simulink library "LopesDevelopmentLibrary"  (R2015b)
settings: Solver=ode45  StartTime=0.0  StopTime=10.0  RelTol=1e-3
values from neighbouring files (symbols this model uses):
  d2r = @(d) d*(pi/180)    [LopesDevelopmentLibrary_LoadParameters.m]
  ts = LopesParams.ts    [LopesDevelopmentLibrary_LoadParameters.m]
undefined symbols (not defined in the file or in its folder): anyParameterChanged, DiscIntNeverNeededParam, gcbh, LHF, LKF, LopesParams, macaddr, mxpcnetworkconfig, mxpcrtudprx, mxpcrtudptx, patientParametersChanged, port, PX, PZ, RHF, RKF, SelectorLOPESInSize, StrideTime_s, Time
undefined symbols (not defined in the file): LopesParamsSendDataArrayLen
libraries: LopesDevelopmentLibrary x288, simulink x98, dspmtrx3 x47, xpciplib x6, xpcnetworkbufferlib x5, dspsigops x4, dspstat3 x3, xpcethernetlib x2, visionstatistics x2, xpcseriallib x2, nmc x1, simulink_extras x1
(part 9 of 12)

== system LopesDevelopmentLibrary/GaitGenerationExtra/CalculateBreaksCoefs/Calculate/RightHipFlexion1 ==
  parameters : Inport
  HipExtensionOffset_pct : Inport  Port=2
  Steplength_Length_pct : Inport  Port=3
  SteplengthOtherLeg_Length_pct : Inport  Port=4
  StepHeight_KneeFlexion_pct : Inport  Port=5
  AddToMatrixColumn : LopesDevelopmentLibrary/Various/AddToMatrixColumn  col=2  minimum=-inf  maximum=inf
  Bias : Bias  Bias=100
  Bias1 : Bias  Bias=100
  Gain1 : Gain  Gain=1/100
  Gain2 : Gain  Gain=1/100
  Gain3 : Gain  Gain=0.01* d2r(2.5)
  Gain4 : Gain  Gain=0.01* d2r(5)
  GainHipExtensionOffset : Gain  Gain=-0.01* d2r(10)
  KneeFlexionStepheight : LopesDevelopmentLibrary/Various/AddToMatrixElement  row=5  col=2  minimum=0  maximum=d2r(90)
  KneeFlexionStepheight1 : LopesDevelopmentLibrary/Various/AddToMatrixElement  row=6  col=2  minimum=0  maximum=d2r(90)
  MultiplyMatrixElement : LopesDevelopmentLibrary/Various/MultiplyMatrixElement  row=6  col=2  minimum=-inf  maximum=inf
  MultiplyMatrixElement1 : LopesDevelopmentLibrary/Various/MultiplyMatrixElement  row=4  col=2  minimum=-inf  maximum=inf
  MultiplyMatrixElement2 : LopesDevelopmentLibrary/Various/MultiplyMatrixElement  row=1  col=2  minimum=-inf  maximum=inf
  MultiplyMatrixElement3 : LopesDevelopmentLibrary/Various/MultiplyMatrixElement  row=2  col=2  minimum=-inf  maximum=inf
  RatioFlexionExtension : Gain
  RegressionData : Constant  Value=LopesParams.GaitData.RHF
  RegressionData2KeyEvents : LopesDevelopmentLibrary/BlocksForInternalUse/GaitGeneration/RegressionData2KeyEvents
  KeyEvents : Outport
  wires:
  MultiplyMatrixElement1/1 -> KeyEvents/1
  AddToMatrixColumn/1 -> MultiplyMatrixElement/1
  Gain2/1 -> MultiplyMatrixElement1/2
  Steplength_Length_pct/1 -> Bias/1
  Bias/1 -> Gain1/1
  Gain1/1 -> MultiplyMatrixElement3/2, MultiplyMatrixElement2/2, MultiplyMatrixElement/2
  Bias1/1 -> Gain2/1
  SteplengthOtherLeg_Length_pct/1 -> RatioFlexionExtension/1
  RegressionData/1 -> RegressionData2KeyEvents/1
  parameters/1 -> RegressionData2KeyEvents/2
  KneeFlexionStepheight/1 -> KneeFlexionStepheight1/1
  RegressionData2KeyEvents/1 -> KneeFlexionStepheight/1
  Gain3/1 -> KneeFlexionStepheight/2
  Gain4/1 -> KneeFlexionStepheight1/2
  StepHeight_KneeFlexion_pct/1 -> Gain4/1, Gain3/1
  HipExtensionOffset_pct/1 -> GainHipExtensionOffset/1
  KneeFlexionStepheight1/1 -> AddToMatrixColumn/1
  GainHipExtensionOffset/1 -> AddToMatrixColumn/2
  RatioFlexionExtension/1 -> Bias1/1
  MultiplyMatrixElement/1 -> MultiplyMatrixElement2/1
  MultiplyMatrixElement2/1 -> MultiplyMatrixElement3/1
  MultiplyMatrixElement3/1 -> MultiplyMatrixElement1/1

== system LopesDevelopmentLibrary/GaitGenerationExtra/CalculateBreaksCoefs/Calculate/RightKneeFlexion1 ==
  parameters : Inport
  StepHeight_KneeFlexion_pct : Inport  Port=2
  Prepositioning_KneeFlexion_pct : Inport  Port=3
  StabilityStance_Kneeflexion_pct : Inport  Port=4
  StepLength_pct : Inport  Port=5
  Constant : Constant  Value=-inf
  Gain1 : Gain  Gain=0.01* d2r(5)
  Gain2 : Gain  Gain=0.01* d2r(10)
  Gain3 : Gain  Gain=0.01* d2r(5)
  Gain4 : Gain  Gain=0.01* d2r(20)
  Gain5 : Gain  Gain=-0.01/3
  KneeFlexionPrepositioning : LopesDevelopmentLibrary/Various/AddToMatrixElement  row=1  col=2  minimum=0  maximum=d2r(90)
  KneefFlexionStepheigh : LopesDevelopmentLibrary/Various/AddToMatrixElement  row=5  col=2  minimum=0  maximum=d2r(90)
  KneefFlexionStepheigh1 : LopesDevelopmentLibrary/Various/AddToMatrixElement  row=6  col=2  minimum=0  maximum=d2r(90)
  KneeflexionStance : LopesDevelopmentLibrary/Various/AddToMatrixElement  row=2  col=2  minimum=0  maximum=d2r(90)
  RatioKey6toKey1 : Gain  Gain=1/2
  RegressionData : Constant  Value=LopesParams.GaitData.RKF
  RegressionData2KeyEvents : LopesDevelopmentLibrary/BlocksForInternalUse/GaitGeneration/RegressionData2KeyEvents
  Saturation : Saturate  UpperLimit=0  LowerLimit=-inf
  Saturation Dynamic : simulink/Discontinuities/Saturation Dynamic  OutMin=[]  OutMax=[]  OutDataTypeStr=Inherit: Same as second input  OutDataType=fixdt(1, 16)  OutScaling=2^-10  DoSatur=off
  SelectorK1 : Selector  NumberOfDimensions=2  InputPortWidth=3  IndexOptions=Index vector (dialog),Index vector (dialog)  Indices=1,2  OutputSizes=1,1
  SelectorK2 : Selector  NumberOfDimensions=2  InputPortWidth=3  IndexOptions=Index vector (dialog),Index vector (dialog)  Indices=2,2  OutputSizes=1,1
  Steplength1 : LopesDevelopmentLibrary/Various/AddToMatrixElement  row=1  col=2  minimum=0  maximum=d2r(90)
  Steplength2 : LopesDevelopmentLibrary/Various/AddToMatrixElement  row=6  col=2  minimum=0  maximum=d2r(90)
  Sum : Sum  Inputs=++|
  Sum1 : Sum  Inputs=-+|
  KeyEvents : Outport
  wires:
  Gain4/1 -> KneefFlexionStepheigh1/2
  KneefFlexionStepheigh1/1 -> KneeFlexionPrepositioning/1
  Gain3/1 -> KneeflexionStance/2
  Gain2/1 -> KneefFlexionStepheigh/2
  StepHeight_KneeFlexion_pct/1 -> Gain2/1, Gain4/1
  KneefFlexionStepheigh/1 -> KneefFlexionStepheigh1/1
  RegressionData2KeyEvents/1 -> KneefFlexionStepheigh/1
  KneeFlexionPrepositioning/1 -> KneeflexionStance/1
  parameters/1 -> RegressionData2KeyEvents/2
  RegressionData/1 -> RegressionData2KeyEvents/1
  Prepositioning_KneeFlexion_pct/1 -> Gain1/1
  StabilityStance_Kneeflexion_pct/1 -> Gain3/1
  Gain1/1 -> KneeFlexionPrepositioning/2
  StepLength_pct/1 -> Saturation/1
  Steplength1/1 -> Steplength2/1
  RatioKey6toKey1/1 -> Steplength2/2
  SelectorK2/1 -> Saturation Dynamic/1
  Constant/1 -> Saturation Dynamic/3
  SelectorK1/1 -> Sum1/1, Sum/1
  Gain5/1 -> Sum/2
  Sum/1 -> Saturation Dynamic/2
  Sum1/1 -> RatioKey6toKey1/1, Steplength1/2
  Saturation Dynamic/1 -> Sum1/2
  Saturation/1 -> Gain5/1
  Steplength2/1 -> KeyEvents/1
  KneeflexionStance/1 -> SelectorK1/1, SelectorK2/1, Steplength1/1

== system LopesDevelopmentLibrary/GaitGenerationExtra/CalculateBreaksCoefs/Calculate/Time1 ==
  note: v = strideLengh * nStridesPerSecond
      |                   = strideLength / nSecondsPerStride
      | strideTime = nSecondsPerStride = strideLength / v
  note: The key event matrix is generated here; it consists
      | of two rows (ie, a key event at 0% and one at 100%),
      | and the start time (=0) and end time. We need to
      | calculate the slope (in s/%) as well to get a straight line.
  WalkingVelocity_m_s : Inport
  BreaksCoefsBus : Inport  Port=2
  Parameters : Inport  Port=3
  CalculateStrideLength : Subsystem
  Constant : Constant  Value=[0,0,nan; 100,nan,nan]
  Gain : Gain  Gain=0.01
  Mux : Mux  Inputs=2
  Overwrite Values : dspmtrx3/Overwrite Values  OverWriteDiag=Submatrix  valFrom2ndIP=Second input port  ConstValue=0  RowSpan=One row  RowStartMode=Index  RowStartIndex=2  RowEndMode=Last  RowEndIndex=1  ColSpan=One column  ColStartMode=Index  ColStartIndex=2  ColEndMode=Last  ColEndIndex=1  DiagSpan=Range of elements  DiagStartMode=Index  DiagStartIndex=2  DiagEndMode=Index  DiagEndIndex=4
  Overwrite Values1 : dspmtrx3/Overwrite Values  OverWriteDiag=Submatrix  valFrom2ndIP=Second input port  ConstValue=0  RowSpan=All rows  RowStartMode=Index  RowStartIndex=2  RowEndMode=Last  RowEndIndex=1  ColSpan=One column  ColStartMode=Last  ColStartIndex=2  ColEndMode=Last  ColEndIndex=1  DiagSpan=Range of elements  DiagStartMode=Index  DiagStartIndex=2  DiagEndMode=Index  DiagEndIndex=4
  SafeDivide : LopesDevelopmentLibrary/Various/SafeDivide  SystemSampleTime=-1
  KeyEvents : Outport
  StrideTime_s : Outport  Port=2
  wires:
  Mux/1 -> Overwrite Values1/2
  Overwrite Values/1 -> Overwrite Values1/1
  Gain/1 -> Mux/2, Mux/1  "slope"
  Constant/1 -> Overwrite Values/1
  SafeDivide/1 -> StrideTime_s/1, Gain/1, Overwrite Values/2  "StrideTime"
  Overwrite Values1/1 -> KeyEvents/1
  BreaksCoefsBus/1 -> CalculateStrideLength/1(BreaksCoefsBus)
  Parameters/1 -> CalculateStrideLength/2(Parameters)
  WalkingVelocity_m_s/1 -> SafeDivide/2
  CalculateStrideLength/1(StrideLength) -> SafeDivide/1

== system LopesDevelopmentLibrary/GaitGenerationExtra/CalculateBreaksCoefs/Calculate/Unactuated DOFS ==

== system LopesDevelopmentLibrary/GaitGenerationExtra/PhaseEstimatorAoyagi_wPI_Extra/EstimatePhaseDirectlyAoyagi/CalculateFullReferenceTrajectory ==
  BreaksCoefs : Inport
  xx : Inport  Port=2
  Enable : EnablePort
  Bus Selector2 : BusSelector  OutputSignals=LHF,LKF,RHF,RKF,StrideTime_s
  Divide{,1,3..4} (4 alike) : Product  Inputs=*/
  Gain : Gain  Gain=0.01
  Terminator{,1,3..4} (4 alike) : Terminator
  ppval_bus_LHF : LopesDevelopmentLibrary/BlocksForInternalUse/GaitGeneration/ppval_bus
  ppval_bus_LKF : LopesDevelopmentLibrary/BlocksForInternalUse/GaitGeneration/ppval_bus
  ppval_bus_RHF : LopesDevelopmentLibrary/BlocksForInternalUse/GaitGeneration/ppval_bus
  ppval_bus_RKF : LopesDevelopmentLibrary/BlocksForInternalUse/GaitGeneration/ppval_bus
  LHF_yy : Outport
  LKF_yy : Outport  Port=2
  RHF_yy : Outport  Port=3
  RKF_yy : Outport  Port=4
  LHF_dydt : Outport  Port=5
  LKF_dydt : Outport  Port=6
  RHF_dydt : Outport  Port=7
  RKF_dydt : Outport  Port=8
  wires:
  xx/1 -> ppval_bus_RHF/1, ppval_bus_RKF/1, ppval_bus_LKF/1, ppval_bus_LHF/1
  BreaksCoefs/1 -> Bus Selector2/1
  ppval_bus_RHF/3 -> Terminator3/1
  ppval_bus_LKF/3 -> Terminator1/1
  ppval_bus_RKF/3 -> Terminator4/1
  ppval_bus_LHF/3 -> Terminator/1
  Divide4/1 -> RKF_dydt/1
  Divide3/1 -> RHF_dydt/1
  Divide1/1 -> LKF_dydt/1
  Divide/1 -> LHF_dydt/1
  Gain/1 -> Divide/2, Divide1/2, Divide3/2, Divide4/2  "dtdx"
  ppval_bus_RKF/2 -> Divide4/1
  ppval_bus_RHF/2 -> Divide3/1
  ppval_bus_LKF/2 -> Divide1/1
  ppval_bus_LHF/2 -> Divide/1
  ppval_bus_RKF/1 -> RKF_yy/1
  ppval_bus_RHF/1 -> RHF_yy/1
  Bus Selector2/1 -> ppval_bus_LHF/2  "<LHF>"
  Bus Selector2/2 -> ppval_bus_LKF/2  "<LKF>"
  Bus Selector2/3 -> ppval_bus_RHF/2  "<RHF>"
  Bus Selector2/4 -> ppval_bus_RKF/2  "<RKF>"
  Bus Selector2/5 -> Gain/1  "<StrideTime_s>"
  ppval_bus_LHF/1 -> LHF_yy/1
  ppval_bus_LKF/1 -> LKF_yy/1

== system LopesDevelopmentLibrary/GaitGenerationExtra/PhaseEstimatorAoyagi_wPI_Extra/PhaseFilterAoyagi/FinalStateFinisher ==
  note: This block is implemented to have a minimum PhasePercRate during the last step
      | In this way, the last step is always finalized
  PhasePercRate : Inport
  FinalState : Inport  Port=2
  Constant : Constant  Value=inf
  Constant1 : Constant  Value=20
  Product : Product  OutDataTypeStr=double
  Saturation : simulink/Discontinuities/Saturation Dynamic  OutMin=[]  OutMax=[]  OutDataTypeStr=Inherit: Same as second input  OutDataType=fixdt(1, 16)  OutScaling=2^-10  DoSatur=off
  PhasePercRateOut : Outport
  wires:
  PhasePercRate/1 -> Saturation/2
  Constant/1 -> Saturation/1
  Constant1/1 -> Product/1
  FinalState/1 -> Product/2
  Saturation/1 -> PhasePercRateOut/1
  Product/1 -> Saturation/3

== system LopesDevelopmentLibrary/GaitGenerationExtra/PhaseEstimatorAoyagi_wPI_Extra/PhaseFilterAoyagi/Wrap_Min50_Plus50 ==
  note: Wraps the input phase such
      | that the output is always
      | in the range -50<=out<50
      | (even if input is negative).
  In : Inport
  Bias : Bias  Bias=50
  Bias1 : Bias  Bias=-50
  Constant1 : Constant  Value=100
  ShiftedPhase1 : Math  Operator=mod  SaturateOnIntegerOverflow=on
  Out : Outport
  wires:
  Bias1/1 -> Out/1
  Bias/1 -> ShiftedPhase1/1
  Constant1/1 -> ShiftedPhase1/2
  In/1 -> Bias/1
  ShiftedPhase1/1 -> Bias1/1

== system LopesDevelopmentLibrary/GaitPhaseDetection/Gait Phase Detection with Wrapper/Data selection/Angle_l ==
  ankle : Inport
  knee : Inport  Port=2
  hip : Inport  Port=3
  Dot Product : DotProduct  InputSameDT=on  OutDataTypeStr=Inherit: Inherit via internal rule
  Sum1 : Sum  Inputs=-+
  Sum2 : Sum  Inputs=+-
  Trigonometric Function : Trigonometry  Operator=acos
  angle_l : Outport
  wires:
  Sum2/1 -> Dot Product/1
  ankle/1 -> Sum2/1
  Sum1/1 -> Dot Product/2
  hip/1 -> Sum1/2
  knee/1 -> Sum2/2, Sum1/1
  Dot Product/1 -> Trigonometric Function/1
  Trigonometric Function/1 -> angle_l/1

== system LopesDevelopmentLibrary/GaitPhaseDetection/Gait Phase Detection with Wrapper/Data selection/Angle_r ==
  ankle : Inport
  knee : Inport  Port=2
  hip : Inport  Port=3
  Dot Product : DotProduct  InputSameDT=on  OutDataTypeStr=Inherit: Inherit via internal rule
  Sum1 : Sum  Inputs=-+
  Sum2 : Sum  Inputs=+-
  Trigonometric Function : Trigonometry  Operator=acos
  angle_r : Outport
  wires:
  Trigonometric Function/1 -> angle_r/1
  Dot Product/1 -> Trigonometric Function/1
  knee/1 -> Sum1/1, Sum2/2
  hip/1 -> Sum1/2
  Sum1/1 -> Dot Product/2
  ankle/1 -> Sum2/1
  Sum2/1 -> Dot Product/1

== system LopesDevelopmentLibrary/GaitPhaseDetection/Gait Phase Detection with Wrapper/LeftLegWalking/Heel strike detection ==
  note: DAL (daling voor stijging)
  ankle_y_dot : Inport
  ankle_x_dot : Inport  Port=2
  " " : simulink/Logic and Bit Operations/Compare To Constant  relop===  const=0  OutDataTypeStr=uint8  ZeroCross=off
  "   " : MinMax
  "        " : simulink/Discrete/Tapped Delay  vinit=0.0  samptime=-1  NumDelays=5  DelayOrder=Oldest  includeCurrent=off
  "               " : DataTypeConversion
  Daldetectie_stijging : simulink/Logic and Bit Operations/Detect Increase  vinit=0.0  InputProcessing=Inherited  OutDataTypeStr=uint8
  Logical Operator : Logic  Inputs=3  AllPortsSameDT=off  OutDataTypeStr=boolean
  Voorwaarde voor stap_3 : simulink/Logic and Bit Operations/Compare To Constant  relop=<  const=0  OutDataTypeStr=uint8  ZeroCross=off
  Heel_strike : Outport
  wires:
  "   "/1 -> " "/1
  "        "/1 -> "   "/1
  Voorwaarde voor stap_3/1 -> Logical Operator/3
  "               "/1 -> "        "/1
  Daldetectie_stijging/1 -> "               "/1, Logical Operator/1
  Logical Operator/1 -> Heel_strike/1
  ankle_y_dot/1 -> Daldetectie_stijging/1
  ankle_x_dot/1 -> Voorwaarde voor stap_3/1
  " "/1 -> Logical Operator/2

== system LopesDevelopmentLibrary/GaitPhaseDetection/Gait Phase Detection with Wrapper/LeftLegWalking/Heel strike_safety ==
  ankle_x_dot : Inport
  belt_speed : Inport  Port=2
  "        " : simulink/Discrete/Tapped Delay  vinit=0  samptime=-1  NumDelays=20  DelayOrder=Oldest  includeCurrent=off
  2-D Mean : visionstatistics/2-D Mean  run=off  reset_popup=None  directionMode=Entire input  dimension=1  treatSBRowAsCol=on  roiEnable=off  roiType=Rectangles  roiPortion=Entire ROI  roiOutput=Individual statistics for each ROI  roiFlag=off  outputDataTypeStr=Inherit: Same as accumulator  outputLastDataTypeStr=Inherit: Same as accumulator  outputMin=[]  outputMax=[]  accumMode=Binary point scaling  accumWordLength=32  accumFracLength=0  accumDataTypeStr=fixdt([],32,0)  accumLastDataTypeStr=fixdt([],32,0)  roundingMode=Floor  overflowMode=off
  Daldetectie_stijging2 : simulink/Logic and Bit Operations/Detect Increase  vinit=0.0  InputProcessing=Inherited  OutDataTypeStr=uint8
  Data Type Conversion2 : DataTypeConversion
  Gain2 : Gain  Gain=-0.95
  Relational Operator : RelationalOperator  Operator=<  OutDataTypeStr=boolean
  Heel_strike_safety : Outport
  wires:
  belt_speed/1 -> Gain2/1
  ankle_x_dot/1 -> "        "/1
  "        "/1 -> 2-D Mean/1
  Relational Operator/1 -> Data Type Conversion2/1
  Data Type Conversion2/1 -> Daldetectie_stijging2/1
  Daldetectie_stijging2/1 -> Heel_strike_safety/1
  2-D Mean/1 -> Relational Operator/1
  Gain2/1 -> Relational Operator/2

== system LopesDevelopmentLibrary/GaitPhaseDetection/Gait Phase Detection with Wrapper/LeftLegWalking/Toe-off detection ==
  ankle_x_dot : Inport
  knee_angle_dot : Inport  Port=2
  Daldetectie_stijging1 : simulink/Logic and Bit Operations/Detect Increase  vinit=0.0  InputProcessing=Inherited  OutDataTypeStr=uint8
  Daldetectie_stijging2 : simulink/Logic and Bit Operations/Detect Increase  vinit=0.0  InputProcessing=Inherited  OutDataTypeStr=uint8
  Data Type Conversion1 : DataTypeConversion
  Gain : Gain  Gain=2
  Logical Operator : Logic  AllPortsSameDT=off  OutDataTypeStr=boolean
  Voorwaarde voor stap_4 : simulink/Logic and Bit Operations/Compare To Constant  relop=>  const=0  OutDataTypeStr=uint8  ZeroCross=off
  Toe_off : Outport
  wires:
  Daldetectie_stijging1/1 -> Gain/1
  Logical Operator/1 -> Data Type Conversion1/1
  Data Type Conversion1/1 -> Daldetectie_stijging1/1
  Voorwaarde voor stap_4/1 -> Logical Operator/1
  Gain/1 -> Toe_off/1
  knee_angle_dot/1 -> Daldetectie_stijging2/1
  Daldetectie_stijging2/1 -> Logical Operator/2
  ankle_x_dot/1 -> Voorwaarde voor stap_4/1

== system LopesDevelopmentLibrary/GaitPhaseDetection/Gait Phase Detection with Wrapper/RightLegWalking/Heel strike detection ==
  note: DAL (daling voor stijging)
  ankle_y_dot : Inport
  ankle_x_dot : Inport  Port=2
  " " : simulink/Logic and Bit Operations/Compare To Constant  relop===  const=0  OutDataTypeStr=uint8  ZeroCross=off
  "   " : MinMax
  "        " : simulink/Discrete/Tapped Delay  vinit=0.0  samptime=-1  NumDelays=5  DelayOrder=Oldest  includeCurrent=off
  "               " : DataTypeConversion
  Daldetectie_stijging : simulink/Logic and Bit Operations/Detect Increase  vinit=0.0  InputProcessing=Inherited  OutDataTypeStr=uint8
  Logical Operator : Logic  Inputs=3  AllPortsSameDT=off  OutDataTypeStr=boolean
  Voorwaarde voor stap_3 : simulink/Logic and Bit Operations/Compare To Constant  relop=<  const=0  OutDataTypeStr=uint8  ZeroCross=off
  Heel_strike : Outport
  wires:
  Daldetectie_stijging/1 -> Logical Operator/1, "               "/1
  "               "/1 -> "        "/1
  Voorwaarde voor stap_3/1 -> Logical Operator/3
  "        "/1 -> "   "/1
  "   "/1 -> " "/1
  Logical Operator/1 -> Heel_strike/1
  ankle_y_dot/1 -> Daldetectie_stijging/1
  ankle_x_dot/1 -> Voorwaarde voor stap_3/1
  " "/1 -> Logical Operator/2

== system LopesDevelopmentLibrary/GaitPhaseDetection/Gait Phase Detection with Wrapper/RightLegWalking/Heel strike_safety ==
  ankle_x_dot : Inport
  belt_speed : Inport  Port=2
  "        " : simulink/Discrete/Tapped Delay  vinit=0  samptime=-1  NumDelays=20  DelayOrder=Oldest  includeCurrent=off
  2-D Mean : visionstatistics/2-D Mean  run=off  reset_popup=None  directionMode=Entire input  dimension=1  treatSBRowAsCol=on  roiEnable=off  roiType=Rectangles  roiPortion=Entire ROI  roiOutput=Individual statistics for each ROI  roiFlag=off  outputDataTypeStr=Inherit: Same as accumulator  outputLastDataTypeStr=Inherit: Same as accumulator  outputMin=[]  outputMax=[]  accumMode=Binary point scaling  accumWordLength=32  accumFracLength=0  accumDataTypeStr=fixdt([],32,0)  accumLastDataTypeStr=fixdt([],32,0)  roundingMode=Floor  overflowMode=off
  Daldetectie_stijging2 : simulink/Logic and Bit Operations/Detect Increase  vinit=0.0  InputProcessing=Inherited  OutDataTypeStr=uint8
  Data Type Conversion2 : DataTypeConversion
  Gain2 : Gain  Gain=-0.95
  Relational Operator : RelationalOperator  Operator=<  OutDataTypeStr=boolean
  Heel_strike_safety : Outport
  wires:
  Daldetectie_stijging2/1 -> Heel_strike_safety/1
  Data Type Conversion2/1 -> Daldetectie_stijging2/1
  Relational Operator/1 -> Data Type Conversion2/1
  "        "/1 -> 2-D Mean/1
  ankle_x_dot/1 -> "        "/1
  2-D Mean/1 -> Relational Operator/1
  belt_speed/1 -> Gain2/1
  Gain2/1 -> Relational Operator/2

== system LopesDevelopmentLibrary/GaitPhaseDetection/Gait Phase Detection with Wrapper/RightLegWalking/Toe-off detection ==
  ankle_x_dot : Inport
  knee_angle_dot : Inport  Port=2
  Daldetectie_stijging1 : simulink/Logic and Bit Operations/Detect Increase  vinit=0.0  InputProcessing=Inherited  OutDataTypeStr=uint8
  Daldetectie_stijging2 : simulink/Logic and Bit Operations/Detect Increase  vinit=0.0  InputProcessing=Inherited  OutDataTypeStr=uint8
  Data Type Conversion1 : DataTypeConversion
  Gain : Gain  Gain=2
  Logical Operator : Logic  AllPortsSameDT=off  OutDataTypeStr=boolean
  Voorwaarde voor stap_4 : simulink/Logic and Bit Operations/Compare To Constant  relop=>  const=0  OutDataTypeStr=uint8  ZeroCross=off
  Toe_off : Outport
  wires:
  Voorwaarde voor stap_4/1 -> Logical Operator/1
  Data Type Conversion1/1 -> Daldetectie_stijging1/1
  Gain/1 -> Toe_off/1
  knee_angle_dot/1 -> Daldetectie_stijging2/1
  Logical Operator/1 -> Data Type Conversion1/1
  Daldetectie_stijging1/1 -> Gain/1
  Daldetectie_stijging2/1 -> Logical Operator/2
  ankle_x_dot/1 -> Voorwaarde voor stap_4/1

== system LopesDevelopmentLibrary/GaitPhaseDetection/Gait Phase Detection with Wrapper/Smart derivative/Filtered derivative ==
  note: This block is a derivative function
      | second order low pass filter with
      | settable zeta and omega.
      | It works for scalars as well as vectors.
      |
      | You can monitor the output from Python
      | by monitoring OutputValue.s[0,:]
  x : Inport
  cut-off (hz) : Inport  Port=2
  Discrete-Time Integrator : DiscreteIntegrator  InitialConditionSetting=State (most efficient)  SampleTime=-1  ICPrevOutput=DiscIntNeverNeededParam  ICPrevScaledInput=DiscIntNeverNeededParam
  Discrete-Time Integrator1 : DiscreteIntegrator  InitialConditionSetting=State (most efficient)  SampleTime=-1  ICPrevOutput=DiscIntNeverNeededParam  ICPrevScaledInput=DiscIntNeverNeededParam
  Gain : Gain  Gain=2*pi
  Product1 : Product  RndMeth=Zero
  Product2 : Product  RndMeth=Zero
  Sum : Sum  Inputs=|+-
  Sum1 : Sum  Inputs=|+-
  omega_sq : Math  Operator=square  SaturateOnIntegerOverflow=on
  two : Constant  Value=2
  zeta : Constant  Value=0.7
  zeta_omega_2 : Product  Inputs=3  RndMeth=Zero
  x_dot : Outport
  wires:
  Discrete-Time Integrator1/1 -> Sum/2
  Product2/1 -> Sum1/2
  zeta_omega_2/1 -> Product2/2
  Product1/1 -> Sum1/1
  Discrete-Time Integrator/1 -> Discrete-Time Integrator1/1, x_dot/1, Product2/1
  two/1 -> zeta_omega_2/1
  Sum/1 -> Product1/1
  cut-off (hz)/1 -> Gain/1
  zeta/1 -> zeta_omega_2/2
  omega_sq/1 -> Product1/2
  x/1 -> Sum/1
  Sum1/1 -> Discrete-Time Integrator/1
  Gain/1 -> omega_sq/1, zeta_omega_2/3

== system LopesDevelopmentLibrary/GaitPhaseDetection/Gait Phase Detection with Wrapper/Smart derivative/Filtered derivative1 ==
  note: This block is a derivative function
      | second order low pass filter with
      | settable zeta and omega.
      | It works for scalars as well as vectors.
      |
      | You can monitor the output from Python
      | by monitoring OutputValue.s[0,:]
  x : Inport
  cut-off (hz) : Inport  Port=2
  Discrete-Time Integrator : DiscreteIntegrator  InitialConditionSetting=State (most efficient)  SampleTime=-1  ICPrevOutput=DiscIntNeverNeededParam  ICPrevScaledInput=DiscIntNeverNeededParam
  Discrete-Time Integrator1 : DiscreteIntegrator  InitialConditionSetting=State (most efficient)  SampleTime=-1  ICPrevOutput=DiscIntNeverNeededParam  ICPrevScaledInput=DiscIntNeverNeededParam
  Gain : Gain  Gain=2*pi
  Product1 : Product  RndMeth=Zero
  Product2 : Product  RndMeth=Zero
  Sum : Sum  Inputs=|+-
  Sum1 : Sum  Inputs=|+-
  omega_sq : Math  Operator=square  SaturateOnIntegerOverflow=on
  two : Constant  Value=2
  zeta : Constant  Value=0.7
  zeta_omega_2 : Product  Inputs=3  RndMeth=Zero
  x_dot : Outport
  wires:
  Gain/1 -> zeta_omega_2/3, omega_sq/1
  Sum1/1 -> Discrete-Time Integrator/1
  x/1 -> Sum/1
  omega_sq/1 -> Product1/2
  zeta/1 -> zeta_omega_2/2
  cut-off (hz)/1 -> Gain/1
  Sum/1 -> Product1/1
  two/1 -> zeta_omega_2/1
  Discrete-Time Integrator/1 -> Product2/1, x_dot/1, Discrete-Time Integrator1/1
  Product1/1 -> Sum1/1
  zeta_omega_2/1 -> Product2/2
  Product2/1 -> Sum1/2
  Discrete-Time Integrator1/1 -> Sum/2

== system LopesDevelopmentLibrary/GaitPhaseDetection/Gait Phase Detection with Wrapper/Smart derivative/Filtered derivative2 ==
  note: This block is a derivative function
      | second order low pass filter with
      | settable zeta and omega.
      | It works for scalars as well as vectors.
      |
      | You can monitor the output from Python
      | by monitoring OutputValue.s[0,:]
  x : Inport
  cut-off (hz) : Inport  Port=2
  Discrete-Time Integrator : DiscreteIntegrator  InitialConditionSetting=State (most efficient)  SampleTime=-1  ICPrevOutput=DiscIntNeverNeededParam  ICPrevScaledInput=DiscIntNeverNeededParam
  Discrete-Time Integrator1 : DiscreteIntegrator  InitialConditionSetting=State (most efficient)  SampleTime=-1  ICPrevOutput=DiscIntNeverNeededParam  ICPrevScaledInput=DiscIntNeverNeededParam
  Gain : Gain  Gain=2*pi
  Product1 : Product  RndMeth=Zero
  Product2 : Product  RndMeth=Zero
  Sum : Sum  Inputs=|+-
  Sum1 : Sum  Inputs=|+-
  omega_sq : Math  Operator=square  SaturateOnIntegerOverflow=on
  two : Constant  Value=2
  zeta : Constant  Value=0.7
  zeta_omega_2 : Product  Inputs=3  RndMeth=Zero
  x_dot : Outport
  wires:
  Discrete-Time Integrator1/1 -> Sum/2
  Product2/1 -> Sum1/2
  zeta_omega_2/1 -> Product2/2
  Product1/1 -> Sum1/1
  Discrete-Time Integrator/1 -> Discrete-Time Integrator1/1, x_dot/1, Product2/1
  two/1 -> zeta_omega_2/1
  Sum/1 -> Product1/1
  cut-off (hz)/1 -> Gain/1
  zeta/1 -> zeta_omega_2/2
  omega_sq/1 -> Product1/2
  x/1 -> Sum/1
  Sum1/1 -> Discrete-Time Integrator/1
  Gain/1 -> omega_sq/1, zeta_omega_2/3

== system LopesDevelopmentLibrary/GaitPhaseDetection/Gait Phase Detection with Wrapper/Smart derivative/Filtered derivative3 ==
  note: This block is a derivative function
      | second order low pass filter with
      | settable zeta and omega.
      | It works for scalars as well as vectors.
      |
      | You can monitor the output from Python
      | by monitoring OutputValue.s[0,:]
  x : Inport
  cut-off (hz) : Inport  Port=2
  Discrete-Time Integrator : DiscreteIntegrator  InitialConditionSetting=State (most efficient)  SampleTime=-1  ICPrevOutput=DiscIntNeverNeededParam  ICPrevScaledInput=DiscIntNeverNeededParam
  Discrete-Time Integrator1 : DiscreteIntegrator  InitialConditionSetting=State (most efficient)  SampleTime=-1  ICPrevOutput=DiscIntNeverNeededParam  ICPrevScaledInput=DiscIntNeverNeededParam
  Gain : Gain  Gain=2*pi
  Product1 : Product  RndMeth=Zero
  Product2 : Product  RndMeth=Zero
  Sum : Sum  Inputs=|+-
  Sum1 : Sum  Inputs=|+-
  omega_sq : Math  Operator=square  SaturateOnIntegerOverflow=on
  two : Constant  Value=2
  zeta : Constant  Value=0.7
  zeta_omega_2 : Product  Inputs=3  RndMeth=Zero
  x_dot : Outport
  wires:
  Gain/1 -> zeta_omega_2/3, omega_sq/1
  Sum1/1 -> Discrete-Time Integrator/1
  x/1 -> Sum/1
  omega_sq/1 -> Product1/2
  zeta/1 -> zeta_omega_2/2
  cut-off (hz)/1 -> Gain/1
  Sum/1 -> Product1/1
  two/1 -> zeta_omega_2/1
  Discrete-Time Integrator/1 -> Product2/1, x_dot/1, Discrete-Time Integrator1/1
  Product1/1 -> Sum1/1
  zeta_omega_2/1 -> Product2/2
  Product2/1 -> Sum1/2
  Discrete-Time Integrator1/1 -> Sum/2

== system LopesDevelopmentLibrary/GaitPhaseDetection/Gait Phase Detection with Wrapper/Smart derivative/Filtered derivative4 ==
  note: This block is a derivative function
      | second order low pass filter with
      | settable zeta and omega.
      | It works for scalars as well as vectors.
      |
      | You can monitor the output from Python
      | by monitoring OutputValue.s[0,:]
  x : Inport
  cut-off (hz) : Inport  Port=2
  Discrete-Time Integrator : DiscreteIntegrator  InitialConditionSetting=State (most efficient)  SampleTime=-1  ICPrevOutput=DiscIntNeverNeededParam  ICPrevScaledInput=DiscIntNeverNeededParam
  Discrete-Time Integrator1 : DiscreteIntegrator  InitialConditionSetting=State (most efficient)  SampleTime=-1  ICPrevOutput=DiscIntNeverNeededParam  ICPrevScaledInput=DiscIntNeverNeededParam
  Gain : Gain  Gain=2*pi
  Product1 : Product  RndMeth=Zero
  Product2 : Product  RndMeth=Zero
  Sum : Sum  Inputs=|+-
  Sum1 : Sum  Inputs=|+-
  omega_sq : Math  Operator=square  SaturateOnIntegerOverflow=on
  two : Constant  Value=2
  zeta : Constant  Value=0.7
  zeta_omega_2 : Product  Inputs=3  RndMeth=Zero
  x_dot : Outport
  wires:
  Discrete-Time Integrator1/1 -> Sum/2
  Product2/1 -> Sum1/2
  zeta_omega_2/1 -> Product2/2
  Product1/1 -> Sum1/1
  Discrete-Time Integrator/1 -> Discrete-Time Integrator1/1, x_dot/1, Product2/1
  two/1 -> zeta_omega_2/1
  Sum/1 -> Product1/1
  cut-off (hz)/1 -> Gain/1
  zeta/1 -> zeta_omega_2/2
  omega_sq/1 -> Product1/2
  x/1 -> Sum/1
  Sum1/1 -> Discrete-Time Integrator/1
  Gain/1 -> omega_sq/1, zeta_omega_2/3

== system LopesDevelopmentLibrary/GaitPhaseDetection/Gait Phase Detection with Wrapper/Smart derivative/Filtered derivative5 ==
  note: This block is a derivative function
      | second order low pass filter with
      | settable zeta and omega.
      | It works for scalars as well as vectors.
      |
      | You can monitor the output from Python
      | by monitoring OutputValue.s[0,:]
  x : Inport
  cut-off (hz) : Inport  Port=2
  Discrete-Time Integrator : DiscreteIntegrator  InitialConditionSetting=State (most efficient)  SampleTime=-1  ICPrevOutput=DiscIntNeverNeededParam  ICPrevScaledInput=DiscIntNeverNeededParam
  Discrete-Time Integrator1 : DiscreteIntegrator  InitialConditionSetting=State (most efficient)  SampleTime=-1  ICPrevOutput=DiscIntNeverNeededParam  ICPrevScaledInput=DiscIntNeverNeededParam
  Gain : Gain  Gain=2*pi
  Product1 : Product  RndMeth=Zero
  Product2 : Product  RndMeth=Zero
  Sum : Sum  Inputs=|+-
  Sum1 : Sum  Inputs=|+-
  omega_sq : Math  Operator=square  SaturateOnIntegerOverflow=on
  two : Constant  Value=2
  zeta : Constant  Value=0.7
  zeta_omega_2 : Product  Inputs=3  RndMeth=Zero
  x_dot : Outport
  wires:
  Gain/1 -> zeta_omega_2/3, omega_sq/1
  Sum1/1 -> Discrete-Time Integrator/1
  x/1 -> Sum/1
  omega_sq/1 -> Product1/2
  zeta/1 -> zeta_omega_2/2
  cut-off (hz)/1 -> Gain/1
  Sum/1 -> Product1/1
  two/1 -> zeta_omega_2/1
  Discrete-Time Integrator/1 -> Product2/1, x_dot/1, Discrete-Time Integrator1/1
  Product1/1 -> Sum1/1
  zeta_omega_2/1 -> Product2/2
  Product2/1 -> Sum1/2
  Discrete-Time Integrator1/1 -> Sum/2

== system LopesDevelopmentLibrary/GaitPhaseDetection/Gait Phase Detection with Wrapper/Smart derivative/belt_speed to cut-off ==
  belt speed : Inport
  Bias : Bias  Bias=1
  Gain : Gain  Gain=26
  Saturation : Saturate  UpperLimit=10  LowerLimit=3
  cut-off (hz) : Outport
  wires:
  Bias/1 -> Saturation/1
  belt speed/1 -> Gain/1
  Gain/1 -> Bias/1
  Saturation/1 -> cut-off (hz)/1

== system LopesDevelopmentLibrary/GaitPhaseDetection/Gait Phase detection/Data selection/Angle_l ==
  ankle : Inport
  knee : Inport  Port=2
  hip : Inport  Port=3
  Dot Product : DotProduct  InputSameDT=on  OutDataTypeStr=Inherit: Inherit via internal rule
  Sum1 : Sum  Inputs=-+
  Sum2 : Sum  Inputs=+-
  Trigonometric Function : Trigonometry  Operator=acos
  angle_l : Outport
  wires:
  Trigonometric Function/1 -> angle_l/1
  Dot Product/1 -> Trigonometric Function/1
  knee/1 -> Sum1/1, Sum2/2
  hip/1 -> Sum1/2
  Sum1/1 -> Dot Product/2
  ankle/1 -> Sum2/1
  Sum2/1 -> Dot Product/1

== system LopesDevelopmentLibrary/GaitPhaseDetection/Gait Phase detection/Data selection/Angle_r ==
  ankle : Inport
  knee : Inport  Port=2
  hip : Inport  Port=3
  Dot Product : DotProduct  InputSameDT=on  OutDataTypeStr=Inherit: Inherit via internal rule
  Sum1 : Sum  Inputs=-+
  Sum2 : Sum  Inputs=+-
  Trigonometric Function : Trigonometry  Operator=acos
  angle_r : Outport
  wires:
  Sum2/1 -> Dot Product/1
  ankle/1 -> Sum2/1
  Sum1/1 -> Dot Product/2
  hip/1 -> Sum1/2
  knee/1 -> Sum2/2, Sum1/1
  Dot Product/1 -> Trigonometric Function/1
  Trigonometric Function/1 -> angle_r/1

== system LopesDevelopmentLibrary/GaitPhaseDetection/Gait Phase detection/LeftLeg/Heel strike detection ==
  note: DAL (daling voor stijging)
  ankle_y_dot : Inport
  ankle_x_dot : Inport  Port=2
  " " : simulink/Logic and Bit Operations/Compare To Constant  relop===  const=0  OutDataTypeStr=uint8  ZeroCross=off
  "   " : MinMax
  "        " : simulink/Discrete/Tapped Delay  vinit=0.0  samptime=-1  NumDelays=5  DelayOrder=Oldest  includeCurrent=off
  "               " : DataTypeConversion
  Daldetectie_stijging : simulink/Logic and Bit Operations/Detect Increase  vinit=0.0  InputProcessing=Inherited  OutDataTypeStr=uint8
  Logical Operator : Logic  Inputs=4  AllPortsSameDT=off  OutDataTypeStr=boolean
  Voorwaarde voor stap_2 : simulink/Logic and Bit Operations/Compare To Constant  relop=<  const=-0.01  OutDataTypeStr=uint8  ZeroCross=off
  Voorwaarde voor stap_3 : simulink/Logic and Bit Operations/Compare To Constant  relop=<  const=0  OutDataTypeStr=uint8  ZeroCross=off
  Heel_strike : Outport
  wires:
  " "/1 -> Logical Operator/4
  "   "/1 -> " "/1
  "        "/1 -> "   "/1
  Voorwaarde voor stap_3/1 -> Logical Operator/3
  "               "/1 -> "        "/1
  Voorwaarde voor stap_2/1 -> Logical Operator/2
  Daldetectie_stijging/1 -> "               "/1, Logical Operator/1
  Logical Operator/1 -> Heel_strike/1
  ankle_x_dot/1 -> Voorwaarde voor stap_3/1
  ankle_y_dot/1 -> Voorwaarde voor stap_2/1, Daldetectie_stijging/1

== system LopesDevelopmentLibrary/GaitPhaseDetection/Gait Phase detection/LeftLeg/Heel strike_safety ==
  ankle_x_dot : Inport
  belt_speed : Inport  Port=2
  "        " : simulink/Discrete/Tapped Delay  vinit=0  samptime=-1  NumDelays=100  DelayOrder=Oldest  includeCurrent=off
  Daldetectie_stijging2 : simulink/Logic and Bit Operations/Detect Increase  vinit=0.0  InputProcessing=Inherited  OutDataTypeStr=uint8
  Data Type Conversion2 : DataTypeConversion
  Gain1 : Gain  Gain=-0.99
  Mean : Subsystem
  Relational Operator : RelationalOperator  Operator=<  OutDataTypeStr=boolean
  Heel_strike_safety : Outport
  wires:
  Gain1/1 -> Relational Operator/2
  belt_speed/1 -> Gain1/1
  Mean/1(Out1) -> Relational Operator/1
  ankle_x_dot/1 -> "        "/1
  "        "/1 -> Mean/1(In1)
  Relational Operator/1 -> Data Type Conversion2/1
  Data Type Conversion2/1 -> Daldetectie_stijging2/1
  Daldetectie_stijging2/1 -> Heel_strike_safety/1

== system LopesDevelopmentLibrary/GaitPhaseDetection/Gait Phase detection/LeftLeg/Toe-off detection ==
  ankle_x_dot : Inport
  knee_angle_dot : Inport  Port=2
  Daldetectie_stijging1 : simulink/Logic and Bit Operations/Detect Increase  vinit=0.0  InputProcessing=Inherited  OutDataTypeStr=uint8
  Daldetectie_stijging2 : simulink/Logic and Bit Operations/Detect Increase  vinit=0.0  InputProcessing=Inherited  OutDataTypeStr=uint8
  Data Type Conversion1 : DataTypeConversion
  Gain : Gain  Gain=2
  Logical Operator : Logic  Inputs=3  AllPortsSameDT=off  OutDataTypeStr=boolean
  Voorwaarde voor stap_1 : simulink/Logic and Bit Operations/Compare To Constant  relop=<  const=9  OutDataTypeStr=uint8  ZeroCross=off
  Voorwaarde voor stap_4 : simulink/Logic and Bit Operations/Compare To Constant  relop=>  const=0  OutDataTypeStr=uint8  ZeroCross=off
  Toe_off : Outport
  wires:
  Voorwaarde voor stap_1/1 -> Logical Operator/3
  knee_angle_dot/1 -> Daldetectie_stijging2/1, Voorwaarde voor stap_1/1
  Daldetectie_stijging1/1 -> Gain/1
  Logical Operator/1 -> Data Type Conversion1/1
  Daldetectie_stijging2/1 -> Logical Operator/2
  Gain/1 -> Toe_off/1
  Data Type Conversion1/1 -> Daldetectie_stijging1/1
  Voorwaarde voor stap_4/1 -> Logical Operator/1
  ankle_x_dot/1 -> Voorwaarde voor stap_4/1

== system LopesDevelopmentLibrary/GaitPhaseDetection/Gait Phase detection/RightLeg/Heel strike detection1 ==
  note: DAL (daling voor stijging)
  ankle_y_dot : Inport
  ankle_x_dot : Inport  Port=2
  " " : simulink/Logic and Bit Operations/Compare To Constant  relop===  const=0  OutDataTypeStr=uint8  ZeroCross=off
  "   " : MinMax
  "        " : simulink/Discrete/Tapped Delay  vinit=0.0  samptime=-1  NumDelays=5  DelayOrder=Oldest  includeCurrent=off
  "               " : DataTypeConversion
  Daldetectie_stijging : simulink/Logic and Bit Operations/Detect Increase  vinit=0.0  InputProcessing=Inherited  OutDataTypeStr=uint8
  Logical Operator : Logic  Inputs=4  AllPortsSameDT=off  OutDataTypeStr=boolean
  Voorwaarde voor stap_2 : simulink/Logic and Bit Operations/Compare To Constant  relop=<  const=-0.01  OutDataTypeStr=uint8  ZeroCross=off
  Voorwaarde voor stap_3 : simulink/Logic and Bit Operations/Compare To Constant  relop=<  const=0  OutDataTypeStr=uint8  ZeroCross=off
  Heel_strike : Outport
  wires:
  " "/1 -> Logical Operator/4
  "   "/1 -> " "/1
  "        "/1 -> "   "/1
  Voorwaarde voor stap_3/1 -> Logical Operator/3
  "               "/1 -> "        "/1
  Voorwaarde voor stap_2/1 -> Logical Operator/2
  Daldetectie_stijging/1 -> "               "/1, Logical Operator/1
  Logical Operator/1 -> Heel_strike/1
  ankle_x_dot/1 -> Voorwaarde voor stap_3/1
  ankle_y_dot/1 -> Voorwaarde voor stap_2/1, Daldetectie_stijging/1

== system LopesDevelopmentLibrary/GaitPhaseDetection/Gait Phase detection/RightLeg/Heel strike_safety1 ==
  ankle_x_dot : Inport
  belt_speed : Inport  Port=2
  "        " : simulink/Discrete/Tapped Delay  vinit=0  samptime=-1  NumDelays=100  DelayOrder=Oldest  includeCurrent=off
  Daldetectie_stijging2 : simulink/Logic and Bit Operations/Detect Increase  vinit=0.0  InputProcessing=Inherited  OutDataTypeStr=uint8
  Data Type Conversion2 : DataTypeConversion
  Gain2 : Gain  Gain=-0.99
  Mean : Subsystem
  Relational Operator : RelationalOperator  Operator=<  OutDataTypeStr=boolean
  Heel_strike_safety : Outport
  wires:
  Gain2/1 -> Relational Operator/2
  belt_speed/1 -> Gain2/1
  Mean/1(Out1) -> Relational Operator/1
  ankle_x_dot/1 -> "        "/1
  "        "/1 -> Mean/1(In1)
  Relational Operator/1 -> Data Type Conversion2/1
  Data Type Conversion2/1 -> Daldetectie_stijging2/1
  Daldetectie_stijging2/1 -> Heel_strike_safety/1

== system LopesDevelopmentLibrary/GaitPhaseDetection/Gait Phase detection/RightLeg/Toe-off detection1 ==
  ankle_x_dot : Inport
  knee_angle_dot : Inport  Port=2
  Daldetectie_stijging1 : simulink/Logic and Bit Operations/Detect Increase  vinit=0.0  InputProcessing=Inherited  OutDataTypeStr=uint8
  Daldetectie_stijging2 : simulink/Logic and Bit Operations/Detect Increase  vinit=0.0  InputProcessing=Inherited  OutDataTypeStr=uint8
  Data Type Conversion1 : DataTypeConversion
  Gain : Gain  Gain=2
  Logical Operator : Logic  Inputs=3  AllPortsSameDT=off  OutDataTypeStr=boolean
  Voorwaarde voor stap_1 : simulink/Logic and Bit Operations/Compare To Constant  relop=<  const=9  OutDataTypeStr=uint8  ZeroCross=off
  Voorwaarde voor stap_4 : simulink/Logic and Bit Operations/Compare To Constant  relop=>  const=0  OutDataTypeStr=uint8  ZeroCross=off
  Toe_off : Outport
  wires:
  Voorwaarde voor stap_1/1 -> Logical Operator/3
  Daldetectie_stijging2/1 -> Logical Operator/2
  Daldetectie_stijging1/1 -> Gain/1
  Logical Operator/1 -> Data Type Conversion1/1
  knee_angle_dot/1 -> Daldetectie_stijging2/1, Voorwaarde voor stap_1/1
  Gain/1 -> Toe_off/1
  Data Type Conversion1/1 -> Daldetectie_stijging1/1
  Voorwaarde voor stap_4/1 -> Logical Operator/1
  ankle_x_dot/1 -> Voorwaarde voor stap_4/1

== system LopesDevelopmentLibrary/GaitPhaseDetection/Gait Phase detection/Smart derivative/Filtered derivative ==
  note: This block is a derivative function
      | second order low pass filter with
      | settable zeta and omega.
      | It works for scalars as well as vectors.
      |
      | You can monitor the output from Python
      | by monitoring OutputValue.s[0,:]
  x : Inport
  cut-off (hz) : Inport  Port=2
  Gain : Gain  Gain=2*pi
  Integrator : Integrator
  Integrator1 : Integrator
  Product1 : Product  RndMeth=Zero
  Product2 : Product  RndMeth=Zero
  Sum : Sum  Inputs=|+-
  Sum1 : Sum  Inputs=|+-
  omega_sq : Math  Operator=square  SaturateOnIntegerOverflow=on
  two : Constant  Value=2
  zeta : Constant  Value=0.7
  zeta_omega_2 : Product  Inputs=3  RndMeth=Zero
  x_dot : Outport
  wires:
  Gain/1 -> zeta_omega_2/3, omega_sq/1
  Sum1/1 -> Integrator/1
  x/1 -> Sum/1
  omega_sq/1 -> Product1/2
  zeta/1 -> zeta_omega_2/2
  cut-off (hz)/1 -> Gain/1
  Sum/1 -> Product1/1
  two/1 -> zeta_omega_2/1
  Integrator/1 -> Product2/1, Integrator1/1, x_dot/1
  Product1/1 -> Sum1/1
  zeta_omega_2/1 -> Product2/2
  Product2/1 -> Sum1/2
  Integrator1/1 -> Sum/2

== system LopesDevelopmentLibrary/GaitPhaseDetection/Gait Phase detection/Smart derivative/Filtered derivative1 ==
  note: This block is a derivative function
      | second order low pass filter with
      | settable zeta and omega.
      | It works for scalars as well as vectors.
      |
      | You can monitor the output from Python
      | by monitoring OutputValue.s[0,:]
  x : Inport
  cut-off (hz) : Inport  Port=2
  Gain : Gain  Gain=2*pi
  Integrator : Integrator
  Integrator1 : Integrator
  Product1 : Product  RndMeth=Zero
  Product2 : Product  RndMeth=Zero
  Sum : Sum  Inputs=|+-
  Sum1 : Sum  Inputs=|+-
  omega_sq : Math  Operator=square  SaturateOnIntegerOverflow=on
  two : Constant  Value=2
  zeta : Constant  Value=0.7
  zeta_omega_2 : Product  Inputs=3  RndMeth=Zero
  x_dot : Outport
  wires:
  Integrator1/1 -> Sum/2
  Product2/1 -> Sum1/2
  zeta_omega_2/1 -> Product2/2
  Product1/1 -> Sum1/1
  Integrator/1 -> x_dot/1, Integrator1/1, Product2/1
  two/1 -> zeta_omega_2/1
  Sum/1 -> Product1/1
  cut-off (hz)/1 -> Gain/1
  zeta/1 -> zeta_omega_2/2
  omega_sq/1 -> Product1/2
  x/1 -> Sum/1
  Sum1/1 -> Integrator/1
  Gain/1 -> omega_sq/1, zeta_omega_2/3

== system LopesDevelopmentLibrary/GaitPhaseDetection/Gait Phase detection/Smart derivative/Filtered derivative2 ==
  note: This block is a derivative function
      | second order low pass filter with
      | settable zeta and omega.
      | It works for scalars as well as vectors.
      |
      | You can monitor the output from Python
      | by monitoring OutputValue.s[0,:]
  x : Inport
  cut-off (hz) : Inport  Port=2
  Gain : Gain  Gain=2*pi
  Integrator : Integrator
  Integrator1 : Integrator
  Product1 : Product  RndMeth=Zero
  Product2 : Product  RndMeth=Zero
  Sum : Sum  Inputs=|+-
  Sum1 : Sum  Inputs=|+-
  omega_sq : Math  Operator=square  SaturateOnIntegerOverflow=on
  two : Constant  Value=2
  zeta : Constant  Value=0.7
  zeta_omega_2 : Product  Inputs=3  RndMeth=Zero
  x_dot : Outport
  wires:
  Gain/1 -> zeta_omega_2/3, omega_sq/1
  Sum1/1 -> Integrator/1
  x/1 -> Sum/1
  omega_sq/1 -> Product1/2
  zeta/1 -> zeta_omega_2/2
  cut-off (hz)/1 -> Gain/1
  Sum/1 -> Product1/1
  two/1 -> zeta_omega_2/1
  Integrator/1 -> Product2/1, Integrator1/1, x_dot/1
  Product1/1 -> Sum1/1
  zeta_omega_2/1 -> Product2/2
  Product2/1 -> Sum1/2
  Integrator1/1 -> Sum/2

== system LopesDevelopmentLibrary/GaitPhaseDetection/Gait Phase detection/Smart derivative/Filtered derivative3 ==
  note: This block is a derivative function
      | second order low pass filter with
      | settable zeta and omega.
      | It works for scalars as well as vectors.
      |
      | You can monitor the output from Python
      | by monitoring OutputValue.s[0,:]
  x : Inport
  cut-off (hz) : Inport  Port=2
  Gain : Gain  Gain=2*pi
  Integrator : Integrator
  Integrator1 : Integrator
  Product1 : Product  RndMeth=Zero
  Product2 : Product  RndMeth=Zero
  Sum : Sum  Inputs=|+-
  Sum1 : Sum  Inputs=|+-
  omega_sq : Math  Operator=square  SaturateOnIntegerOverflow=on
  two : Constant  Value=2
  zeta : Constant  Value=0.7
  zeta_omega_2 : Product  Inputs=3  RndMeth=Zero
  x_dot : Outport
  wires:
  Integrator1/1 -> Sum/2
  Product2/1 -> Sum1/2
  zeta_omega_2/1 -> Product2/2
  Product1/1 -> Sum1/1
  Integrator/1 -> x_dot/1, Integrator1/1, Product2/1
  two/1 -> zeta_omega_2/1
  Sum/1 -> Product1/1
  cut-off (hz)/1 -> Gain/1
  zeta/1 -> zeta_omega_2/2
  omega_sq/1 -> Product1/2
  x/1 -> Sum/1
  Sum1/1 -> Integrator/1
  Gain/1 -> omega_sq/1, zeta_omega_2/3

== system LopesDevelopmentLibrary/GaitPhaseDetection/Gait Phase detection/Smart derivative/Filtered derivative4 ==
  note: This block is a derivative function
      | second order low pass filter with
      | settable zeta and omega.
      | It works for scalars as well as vectors.
      |
      | You can monitor the output from Python
      | by monitoring OutputValue.s[0,:]
  x : Inport
  cut-off (hz) : Inport  Port=2
  Gain : Gain  Gain=2*pi
  Integrator : Integrator
  Integrator1 : Integrator
  Product1 : Product  RndMeth=Zero
  Product2 : Product  RndMeth=Zero
  Sum : Sum  Inputs=|+-
  Sum1 : Sum  Inputs=|+-
  omega_sq : Math  Operator=square  SaturateOnIntegerOverflow=on
  two : Constant  Value=2
  zeta : Constant  Value=0.7
  zeta_omega_2 : Product  Inputs=3  RndMeth=Zero
  x_dot : Outport
  wires:
  Integrator1/1 -> Sum/2
  Product2/1 -> Sum1/2
  zeta_omega_2/1 -> Product2/2
  Product1/1 -> Sum1/1
  Integrator/1 -> x_dot/1, Integrator1/1, Product2/1
  two/1 -> zeta_omega_2/1
  Sum/1 -> Product1/1
  cut-off (hz)/1 -> Gain/1
  zeta/1 -> zeta_omega_2/2
  omega_sq/1 -> Product1/2
  x/1 -> Sum/1
  Sum1/1 -> Integrator/1
  Gain/1 -> omega_sq/1, zeta_omega_2/3

== system LopesDevelopmentLibrary/GaitPhaseDetection/Gait Phase detection/Smart derivative/Filtered derivative5 ==
  note: This block is a derivative function
      | second order low pass filter with
      | settable zeta and omega.
      | It works for scalars as well as vectors.
      |
      | You can monitor the output from Python
      | by monitoring OutputValue.s[0,:]
  x : Inport
  cut-off (hz) : Inport  Port=2
  Gain : Gain  Gain=2*pi
  Integrator : Integrator
  Integrator1 : Integrator
  Product1 : Product  RndMeth=Zero
  Product2 : Product  RndMeth=Zero
  Sum : Sum  Inputs=|+-
  Sum1 : Sum  Inputs=|+-
  omega_sq : Math  Operator=square  SaturateOnIntegerOverflow=on
  two : Constant  Value=2
  zeta : Constant  Value=0.7
  zeta_omega_2 : Product  Inputs=3  RndMeth=Zero
  x_dot : Outport
  wires:
  Gain/1 -> zeta_omega_2/3, omega_sq/1
  Sum1/1 -> Integrator/1
  x/1 -> Sum/1
  omega_sq/1 -> Product1/2
  zeta/1 -> zeta_omega_2/2
  cut-off (hz)/1 -> Gain/1
  Sum/1 -> Product1/1
  two/1 -> zeta_omega_2/1
  Integrator/1 -> Product2/1, Integrator1/1, x_dot/1
  Product1/1 -> Sum1/1
  zeta_omega_2/1 -> Product2/2
  Product2/1 -> Sum1/2
  Integrator1/1 -> Sum/2

== system LopesDevelopmentLibrary/GaitPhaseDetection/Gait Phase detection/Smart derivative/belt_speed to cut-off ==
  belt speed : Inport
  Bias : Bias  Bias=1
  Gain : Gain  Gain=26
  Saturation : Saturate  UpperLimit=10  LowerLimit=3
  cut-off (hz) : Outport
  wires:
  Saturation/1 -> cut-off (hz)/1
  Gain/1 -> Bias/1
  belt speed/1 -> Gain/1
  Bias/1 -> Saturation/1

== system LopesDevelopmentLibrary/Mindwalker/Mindwalker_Lopes_Conversion/CalculateForceOnTorso/CalculateDampingTerm ==
  note: Stiffness may be a vector.
  note: If stiffness is a vector,
      | Inertia may be a vector (but scalar is okay too)
  Stiffness : Inport
  Inertia : Inport  Port=2
  DampingCoef : Constant  Value=0.707
  Divide1 : Product  Inputs=*/
  OverrideInertia : Constant  Value=1.5
  Product1 : Product  Inputs=3  RndMeth=Zero
  Sqrt : Sqrt  SaturateOnIntegerOverflow=on
  Switch : Switch  Criteria=u2 ~= 0
  Two : Constant  Value=2
  Damping : Outport
  wires:
  Switch/1 -> Divide1/2
  OverrideInertia/1 -> Switch/1, Switch/2
  DampingCoef/1 -> Product1/1
  Two/1 -> Product1/2
  Sqrt/1 -> Product1/3
  Divide1/1 -> Sqrt/1
  Stiffness/1 -> Divide1/1
  Inertia/1 -> Switch/3
  Product1/1 -> Damping/1

== system LopesDevelopmentLibrary/Mindwalker/Mindwalker_Lopes_Conversion/TorsoDynamics/EndStops ==
  TorsoPos : Inport
  TorsoVel : Inport  Port=2
  TorsoInertia : Inport  Port=3
  Add : Sum
  Add1 : Sum
  Add2 : Sum
  CalculateDampingTerm : Subsystem
  Compare To Zero : simulink/Logic and Bit Operations/Compare To Zero  relop=>=  OutDataTypeStr=boolean
  Compare To Zero1 : simulink/Logic and Bit Operations/Compare To Zero  relop=<=  OutDataTypeStr=boolean
  Data Type Conversion : DataTypeConversion
  Data Type Conversion1 : DataTypeConversion
  HighEndStop_rad : Constant  Value=0.3
  LowwEndStop_rad : Constant  Value=-0.3
  Product{,1..5} (6 alike) : Product  RndMeth=Zero
  Stiffness_Nm_rad : Constant  Value=1000
  Subtract : Sum  Inputs=+-
  Subtract1 : Sum  Inputs=+-
  Unary Minus : UnaryMinus
  Unary Minus1 : UnaryMinus
  EndstopForce : Outport
  wires:
  LowwEndStop_rad/1 -> Subtract1/2
  Subtract1/1 -> Product3/1, Compare To Zero1/1
  Compare To Zero1/1 -> Data Type Conversion1/1
  Stiffness_Nm_rad/1 -> Product/2, Product3/2, CalculateDampingTerm/1(Stiffness)
  CalculateDampingTerm/1(Damping) -> Product1/2, Product4/2
  Product3/1 -> Add1/1
  Product4/1 -> Add1/2
  Add1/1 -> Unary Minus1/1
  Data Type Conversion1/1 -> Product5/1
  Unary Minus1/1 -> Product5/2
  Add/1 -> Unary Minus/1
  TorsoPos/1 -> Subtract/1, Subtract1/1
  TorsoInertia/1 -> CalculateDampingTerm/2(Inertia)
  TorsoVel/1 -> Product1/1, Product4/1
  Product2/1 -> Add2/1
  Product5/1 -> Add2/2
  Add2/1 -> EndstopForce/1
  Product1/1 -> Add/2
  Data Type Conversion/1 -> Product2/1
  Product/1 -> Add/1
  Unary Minus/1 -> Product2/2
  Subtract/1 -> Compare To Zero/1, Product/1
  HighEndStop_rad/1 -> Subtract/2
  Compare To Zero/1 -> Data Type Conversion/1

== system LopesDevelopmentLibrary/Mindwalker/Mindwalker_Lopes_Conversion/TorsoDynamics/TorsoSpring ==
  TorsoPos : Inport
  TorsoVel : Inport  Port=2
  TorsoInertia : Inport  Port=3
  Add : Sum
  CalculateDampingTerm : Subsystem
  Product : Product  RndMeth=Zero
  Product1 : Product  RndMeth=Zero
  Rate Limiter : RateLimiter  RisingSlewLimit=0.1  FallingSlewLimit=-0.1  SampleTimeMode=inherited
  SpringPos : Constant  Value=0
  Stiffness_Nm_rad : Constant  Value=0
  Subtract : Sum  Inputs=+-
  Unary Minus : UnaryMinus
  Force : Outport
  wires:
  Rate Limiter/1 -> Subtract/2
  SpringPos/1 -> Rate Limiter/1
  Subtract/1 -> Product/1
  Product/1 -> Add/1
  Product1/1 -> Add/2
  Unary Minus/1 -> Force/1
  TorsoVel/1 -> Product1/1
  TorsoInertia/1 -> CalculateDampingTerm/2(Inertia)
  TorsoPos/1 -> Subtract/1
  Add/1 -> Unary Minus/1
  CalculateDampingTerm/1(Damping) -> Product1/2
  Stiffness_Nm_rad/1 -> CalculateDampingTerm/1(Stiffness), Product/2
